simulink model "Model_Guido_v2"  (R2020a)
settings: Solver=FixedStepAuto  StartTime=0.0  StopTime=40  RelTol=1e-3
undefined symbols (not defined in the file): Bv, Bvn, Bw, Cv, Cvn, Cw, d, DiscIntNeverNeededParam, J, K_fsfb, K_int, Kt, l, M, r, T_loc, T_odom, Ti, Ts
libraries: simulink x3
settings Model: Creator=User  LastModifiedBy=User
settings SolverCC: ZeroCrossControl=EnableAll  ZeroCrossAlgorithm=Adaptive
settings DebuggingCC: IgnoredZcDiagnostic=none

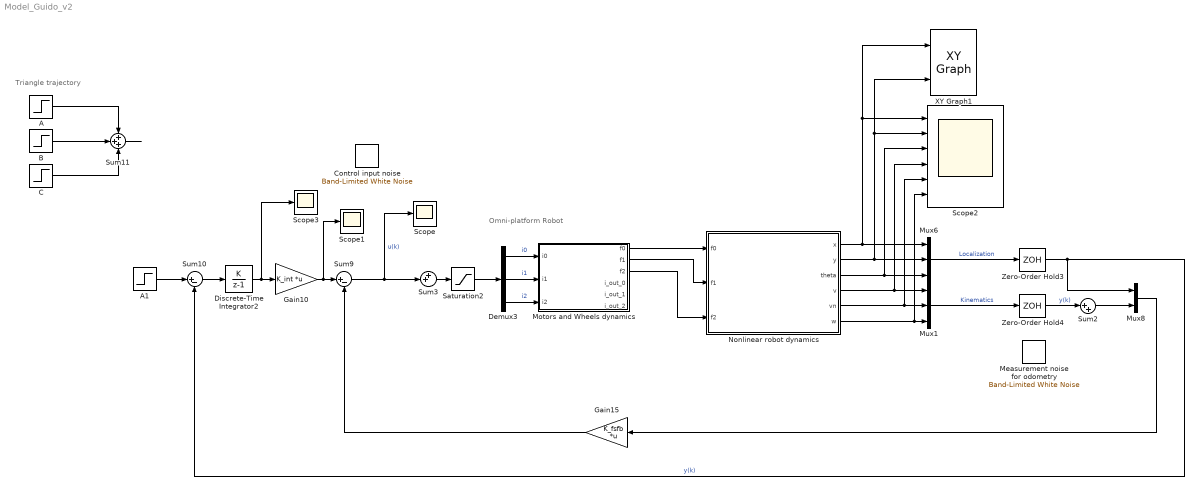
== system Model_Guido_v2 ==
  note: Omni-platform Robot
  note: Triangle trajectory
  A : Step  Time=0  Before=[0 0 0]  After=[0.5 -sqrt(3)/2 1]  SampleTime=Ts
  A1 : Step  Time=0  Before=[0 0 0]  After=[0.1 0 0]
  B : Step  Time=6  Before=[0 0 0]  After=[-1 0 1]  SampleTime=Ts
  C : Step  Time=12  Before=[0 0 0]  After=[0.5 sqrt(3)/2 0]  SampleTime=Ts
  Control input noise : simulink/Sources/Band-Limited White Noise  Cov=[0.001 0.001 0.001]  Ts=Ts  seed=[23341]
  Demux3 : Demux  Outputs=3
  Discrete-Time Integrator2 : DiscreteIntegrator  IntegratorMethod=Accumulation: Forward Euler  InitialCondition=[ 0 0 0]  SampleTime=Ts  ICPrevOutput=DiscIntNeverNeededParam  ICPrevScaledInput=DiscIntNeverNeededParam
  Gain10 : Gain  Gain=K_int  Multiplication=Matrix(K*u) (u vector)
  Gain15 : Gain  Gain=K_fsfb  Multiplication=Matrix(K*u) (u vector)
  Measurement noise for odometry : simulink/Sources/Band-Limited White Noise  Cov=[0.01 0.01 0.01]  Ts=T_odom  seed=[23341]
  "Motors and Wheels dynamics " : Subsystem
  Mux1 : Mux  Inputs=3
  Mux6 : Mux  Inputs=3
  Mux8 : Mux  Inputs=2
  Nonlinear robot dynamics : Subsystem
  Saturation2 : Saturate  UpperLimit=4  LowerLimit=-4
  Scope : Scope
  Scope1 : Scope
  Scope2 : Scope  NumInputPorts=6
  Scope3 : Scope
  Sum10 : Sum  Inputs=|+-
  Sum11 : Sum  Inputs=+++
  Sum2 : Sum  Inputs=|++
  Sum3 : Sum  Inputs=++|
  Sum9 : Sum  Inputs=|+-
  XY Graph1 : simulink/Sinks/XY Graph  xmin=-2  xmax=2  ymin=-2  ymax=2  st=-1
  Zero-Order Hold3 : ZeroOrderHold  SampleTime=T_loc
  Zero-Order Hold4 : ZeroOrderHold  SampleTime=T_odom
  wires:
  Nonlinear robot dynamics/1(x) -> XY Graph1/1, Scope2/1, Mux6/1
  Nonlinear robot dynamics/2(y) -> XY Graph1/2, Scope2/2, Mux6/2
  Nonlinear robot dynamics/3(theta) -> Scope2/3, Mux6/3
  Mux6/1 -> Zero-Order Hold3/1  "Localization"
  C/1 -> Sum11/3
  Sum9/1 -> Sum3/2, Scope/1  "u(k)"
  Zero-Order Hold3/1 -> Mux8/1, Sum10/2  "y(k)"
  Discrete-Time Integrator2/1 -> Scope3/1, Gain10/1
  Sum10/1 -> Discrete-Time Integrator2/1
  Gain15/1 -> Sum9/2
  A/1 -> Sum11/1
  B/1 -> Sum11/2
  Nonlinear robot dynamics/5(vn) -> Mux1/2, Scope2/5
  Nonlinear robot dynamics/6(w) -> Mux1/3, Scope2/6
  Nonlinear robot dynamics/4(v) -> Mux1/1, Scope2/4
  Saturation2/1 -> Demux3/1
  Sum11/1 -> ?
  Demux3/1 -> "Motors and Wheels dynamics "/1(i0)  "i0"
  Demux3/2 -> "Motors and Wheels dynamics "/2(i1)  "i1"
  Demux3/3 -> "Motors and Wheels dynamics "/3(i2)  "i2"
  "Motors and Wheels dynamics "/1(f0) -> Nonlinear robot dynamics/1(f0)
  "Motors and Wheels dynamics "/2(f1) -> Nonlinear robot dynamics/2(f1)
  "Motors and Wheels dynamics "/3(f2) -> Nonlinear robot dynamics/3(f2)
  Zero-Order Hold4/1 -> Sum2/1  "y(k)"
  Mux1/1 -> Zero-Order Hold4/1  "Kinematics"
  Sum2/1 -> Mux8/2
  Sum3/1 -> Saturation2/1
  Mux8/1 -> Gain15/1
  A1/1 -> Sum10/1
  Gain10/1 -> Scope1/1, Sum9/1

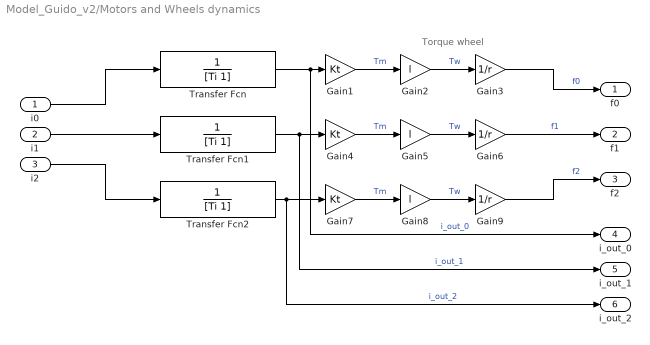
== system Model_Guido_v2/Motors and Wheels dynamics  ==
  note: Torque wheel
  i0 : Inport
  i1 : Inport  Port=2
  i2 : Inport  Port=3
  Gain1 : Gain  Gain=Kt
  Gain2 : Gain  Gain=l
  Gain3 : Gain  Gain=1/r
  Gain4 : Gain  Gain=Kt
  Gain5 : Gain  Gain=l
  Gain6 : Gain  Gain=1/r
  Gain7 : Gain  Gain=Kt
  Gain8 : Gain  Gain=l
  Gain9 : Gain  Gain=1/r
  Transfer Fcn : TransferFcn  Denominator=[Ti 1]
  Transfer Fcn1 : TransferFcn  Denominator=[Ti 1]
  Transfer Fcn2 : TransferFcn  Denominator=[Ti 1]
  f0 : Outport
  f1 : Outport  Port=2
  f2 : Outport  Port=3
  i_out_0 : Outport  Port=4
  i_out_1 : Outport  Port=5
  i_out_2 : Outport  Port=6
  wires:
  i1/1 -> Transfer Fcn1/1
  Gain1/1 -> Gain2/1  "Tm"
  Gain8/1 -> Gain9/1  "Tw"
  Gain5/1 -> Gain6/1  "Tw"
  Transfer Fcn/1 -> i_out_0/1, Gain1/1  "i_out_0"
  Transfer Fcn2/1 -> i_out_2/1, Gain7/1  "i_out_2"
  i2/1 -> Transfer Fcn2/1
  Gain2/1 -> Gain3/1  "Tw"
  Gain7/1 -> Gain8/1  "Tm"
  Transfer Fcn1/1 -> i_out_1/1, Gain4/1  "i_out_1"
  Gain4/1 -> Gain5/1  "Tm"
  Gain3/1 -> f0/1  "f0"
  Gain6/1 -> f1/1  "f1"
  i0/1 -> Transfer Fcn/1
  Gain9/1 -> f2/1  "f2"

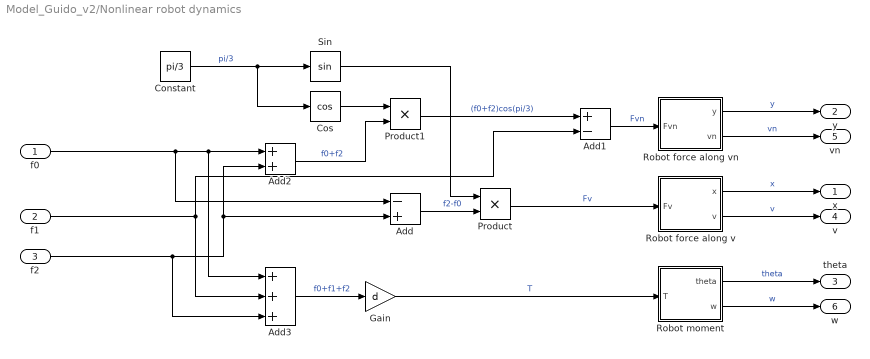
== system Model_Guido_v2/Nonlinear robot dynamics ==
  f0 : Inport
  f1 : Inport  Port=2
  f2 : Inport  Port=3
  Add : Sum  Inputs=-+
  Add1 : Sum  Inputs=+-  AccumDataTypeStr=single  OutDataTypeStr=double
  Add2 : Sum
  Add3 : Sum  Inputs=+++
  Constant : Constant  Value=pi/3
  Cos : Trigonometry  Operator=cos
  Gain : Gain  Gain=d
  Product : Product
  Product1 : Product
  Robot force along v : Subsystem
  Robot force along vn : Subsystem
  Robot moment : Subsystem
  Sin : Trigonometry
  x : Outport
  y : Outport  Port=2
  theta : Outport  Port=3
  v : Outport  Port=4
  vn : Outport  Port=5
  w : Outport  Port=6
  wires:
  f2/1 -> Add3/3, Add2/2, Add/2
  Product1/1 -> Add1/1  "(f0+f2)cos(pi/3)"
  f0/1 -> Add/1, Add3/1, Add2/1
  Cos/1 -> Product1/1
  Product/1 -> Robot force along v/1(Fv)  "Fv"
  Sin/1 -> Product/1
  f1/1 -> Add1/2, Add3/2
  Add2/1 -> Product1/2  "f0+f2"
  Constant/1 -> Cos/1, Sin/1  "pi/3"
  Add/1 -> Product/2  "f2-f0"
  Gain/1 -> Robot moment/1(T)  "T"
  Robot force along vn/1(y) -> y/1  "y"
  Add1/1 -> Robot force along vn/1(Fvn)  "Fvn"
  Add3/1 -> Gain/1  "f0+f1+f2"
  Robot moment/1(theta) -> theta/1  "theta"
  Robot force along v/2(v) -> v/1  "v"
  Robot force along v/1(x) -> x/1  "x"
  Robot moment/2(w) -> w/1  "w"
  Robot force along vn/2(vn) -> vn/1  "vn"

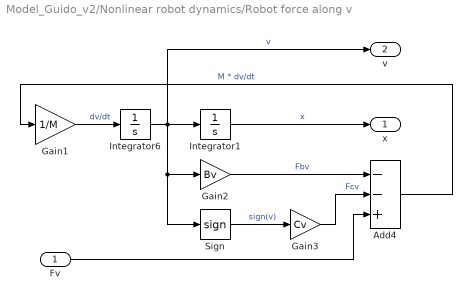
== system Model_Guido_v2/Nonlinear robot dynamics/Robot force along v ==
  Fv : Inport
  Add4 : Sum  Inputs=--+
  Gain1 : Gain  Gain=1/M
  Gain2 : Gain  Gain=Bv
  Gain3 : Gain  Gain=Cv
  Integrator1 : Integrator  ContinuousStateAttributes='x'
  Integrator6 : Integrator  ContinuousStateAttributes='v'
  Sign : Signum
  x : Outport
  v : Outport  Port=2
  wires:
  Fv/1 -> Add4/3
  Sign/1 -> Gain3/1  "sign(v)"
  Gain2/1 -> Add4/1  "Fbv"
  Gain3/1 -> Add4/2  "Fcv"
  Integrator1/1 -> x/1  "x"
  Integrator6/1 -> v/1, Integrator1/1, Sign/1, Gain2/1  "v"
  Gain1/1 -> Integrator6/1  "dv/dt"
  Add4/1 -> Gain1/1  "M * dv/dt"

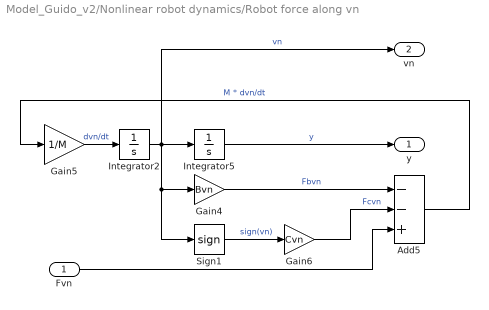
== system Model_Guido_v2/Nonlinear robot dynamics/Robot force along vn ==
  Fvn : Inport
  Add5 : Sum  Inputs=--+
  Gain4 : Gain  Gain=Bvn
  Gain5 : Gain  Gain=1/M
  Gain6 : Gain  Gain=Cvn
  Integrator2 : Integrator  ContinuousStateAttributes='vn'
  Integrator5 : Integrator  ContinuousStateAttributes='y'
  Sign1 : Signum
  y : Outport
  vn : Outport  Port=2
  wires:
  Gain5/1 -> Integrator2/1  "dvn/dt"
  Integrator2/1 -> vn/1, Integrator5/1, Sign1/1, Gain4/1  "vn"
  Gain6/1 -> Add5/2  "Fcvn"
  Fvn/1 -> Add5/3
  Add5/1 -> Gain5/1  "M * dvn/dt"
  Sign1/1 -> Gain6/1  "sign(vn)"
  Gain4/1 -> Add5/1  "Fbvn"
  Integrator5/1 -> y/1  "y"

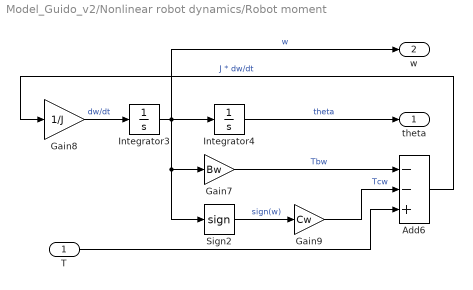
== system Model_Guido_v2/Nonlinear robot dynamics/Robot moment ==
  T : Inport
  Add6 : Sum  Inputs=--+
  Gain7 : Gain  Gain=Bw
  Gain8 : Gain  Gain=1/J
  Gain9 : Gain  Gain=Cw
  Integrator3 : Integrator  ContinuousStateAttributes='w'
  Integrator4 : Integrator  ContinuousStateAttributes='theta'
  Sign2 : Signum
  theta : Outport
  w : Outport  Port=2
  wires:
  Integrator3/1 -> w/1, Integrator4/1, Sign2/1, Gain7/1  "w"
  Gain8/1 -> Integrator3/1  "dw/dt"
  Add6/1 -> Gain8/1  "J * dw/dt"
  Gain9/1 -> Add6/2  "Tcw"
  Gain7/1 -> Add6/1  "Tbw"
  Sign2/1 -> Gain9/1  "sign(w)"
  Integrator4/1 -> theta/1  "theta"
  T/1 -> Add6/3
